simulink model "BBrakeLight"  (R2024b)
settings: configuration reference "STM32H7_Config" (kept outside this file)
libraries: simulink x2
settings Model: DataDictionary=Master_Dictionary.sldd  EnableAccessToBaseWorkspace=off  Creator=torni  LastModifiedBy=William
settings ConfigSetRef: SourceName=STM32H7_Config

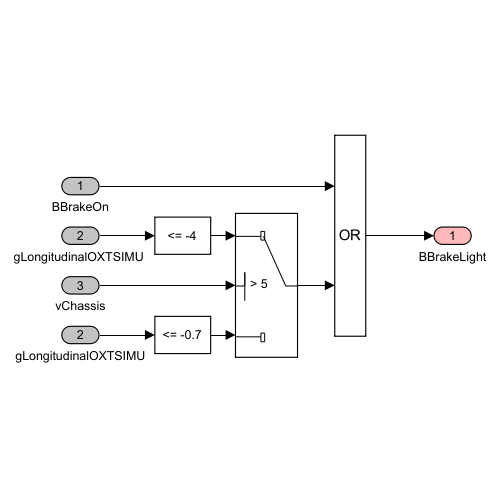
[thumbnail: Simulink's stored preview of the top-level diagram]
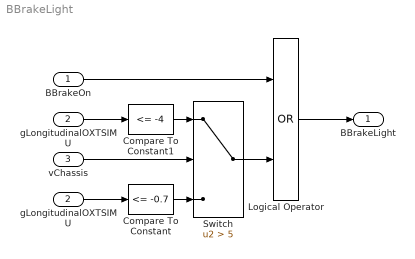
== system BBrakeLight ==
  BBrakeOn : Inport  OutDataTypeStr=boolean
  gLongitudinalOXTSIMU : Inport  Port=2  OutDataTypeStr=double
  vChassis : Inport  Port=3  OutDataTypeStr=double
  Compare To Constant : simulink/Logic and Bit Operations/Compare To Constant  relop=<=  const=-0.7  OutDataTypeStr=boolean
  Compare To Constant1 : simulink/Logic and Bit Operations/Compare To Constant  relop=<=  const=-4  OutDataTypeStr=boolean
  Logical Operator : Logic  Operator=OR  AllPortsSameDT=off  OutDataTypeStr=boolean
  Switch : Switch  Criteria=u2 > Threshold  Threshold=5  SaturateOnIntegerOverflow=off  InputSameDT=off
  "gLongitudinalOXTSIMU " : InportShadow  Port=2  OutDataTypeStr=double
  BBrakeLight : Outport  OutDataTypeStr=boolean  VectorParamsAs1DForOutWhenUnconnected=off
  wires:
  BBrakeOn/1 -> Logical Operator/1
  Logical Operator/1 -> BBrakeLight/1
  gLongitudinalOXTSIMU/1 -> Compare To Constant/1
  Compare To Constant/1 -> Switch/3
  vChassis/1 -> Switch/2
  Switch/1 -> Logical Operator/2
  Compare To Constant1/1 -> Switch/1
  "gLongitudinalOXTSIMU "/1 -> Compare To Constant1/1
